simulink model "simu11_08_14"  (R2014a)
settings: Solver=ode45  StartTime=0.0  StopTime=400  RelTol=1e-3
settings Model: Creator=Cristian  LastModifiedBy=Cristian

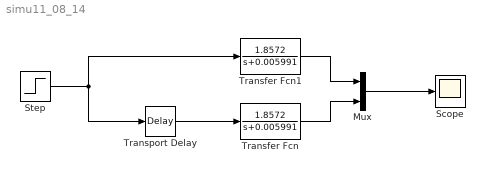
== system simu11_08_14 ==
  Mux : Mux  Inputs=2
  Scope : Scope
  Step : Step  SampleTime=0
  Transfer Fcn : TransferFcn  Numerator=[1.8572]  Denominator=[1 0.005991]
  Transfer Fcn1 : TransferFcn  Numerator=[1.8572]  Denominator=[1 0.005991]
  Transport Delay : TransportDelay  DelayTime=9
  wires:
  Transport Delay/1 -> Transfer Fcn/1
  Step/1 -> Transport Delay/1, Transfer Fcn1/1
  Transfer Fcn/1 -> Mux/2
  Transfer Fcn1/1 -> Mux/1
  Mux/1 -> Scope/1
